simulink model "sim_ES01_03"  (R2021b)
settings: Solver=VariableStepAuto  StartTime=0.0  StopTime=Ts  MaxStep=1e-02  RelTol=1e-3
values from neighbouring files (symbols this model uses):
  c = 2664    [DatiSospensione.m]    (also in Dati_Necessari.m; ES01_Comfort_4dof_stud.m = 0.00047; ES2_2DOF.m = C_values(count2); ES_2DOF_ANIM_TF.m = c_opt)
  k = 35495    [DatiSospensione.m]    (also in Dati_Necessari.m = 99000; ES2_2DOF.m = 99000)
  m = ms+mu    (= 395)    [DatiSospensione.m]    (also in ES01_Comfort_4dof_stud.m = 1790)
  T_sampling = 1/f_sampling    (= 0.001)    [Dati_Necessari.m]    (also in ES_2DOF_ANIM_TF.m)
  Ts = 4    [DatiSospensione.m]    (also in ES_2DOF_ANIM_TF.m = 100)
  z0 = 0    [Dati_Necessari.m]    (also in ES_2DOF_ANIM_TF.m)
  zd0 = 0    [Dati_Necessari.m]    (also in ES_2DOF_ANIM_TF.m)
libraries: simulink x1
settings Model: Creator=Utente  LastModifiedBy=Utente
settings DataIOCC: ReturnWorkspaceOutputs=off

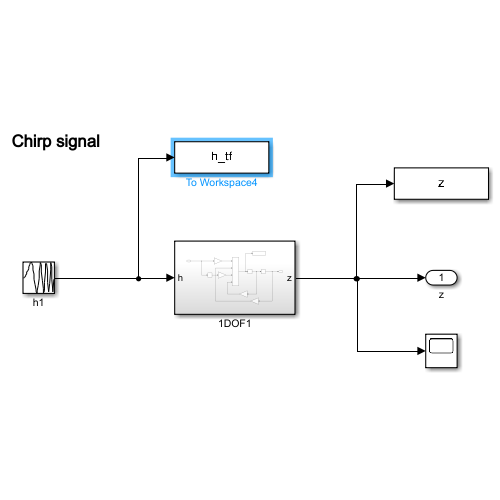
[thumbnail: Simulink's stored preview of the top-level diagram]
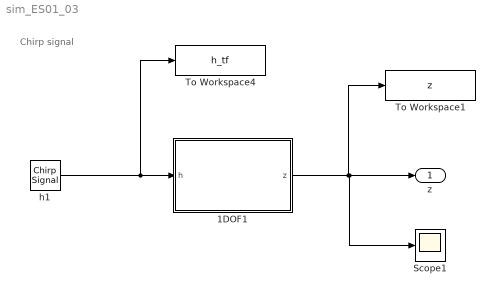
== system sim_ES01_03 ==
  note: Chirp signal
  1DOF1 : Subsystem
  Scope1 : Scope
  To Workspace1 : ToWorkspace  VariableName=z  SaveFormat=Timeseries  SampleTime=1/T_sampling
  To Workspace4 : ToWorkspace  VariableName=h_tf  SaveFormat=Timeseries  SampleTime=1/T_sampling
      settings: Decimation=decimation
  h1 : simulink/Sources/Chirp Signal  f1=w_in  T=Ts  f2=w_end
  z : Outport
  wires:
  h1/1 -> To Workspace4/1, 1DOF1/1(h)
  1DOF1/1(z) -> To Workspace1/1, Scope1/1, z/1

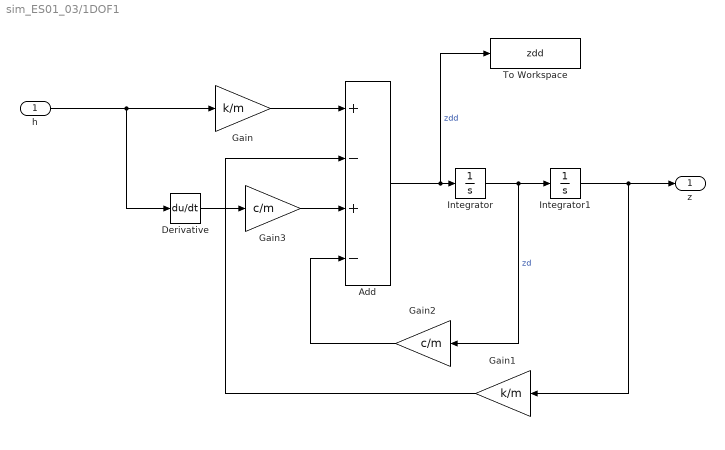
== system sim_ES01_03/1DOF1 ==
  h : Inport
  Add : Sum  Inputs=+-+-
  Derivative : Derivative
  Gain : Gain  Gain=k/m
  Gain1 : Gain  Gain=k/m
  Gain2 : Gain  Gain=c/m
  Gain3 : Gain  Gain=c/m
  Integrator : Integrator  InitialCondition=zd0
  Integrator1 : Integrator  InitialCondition=z0
  To Workspace : ToWorkspace  VariableName=zdd  SaveFormat=Timeseries  SampleTime=1/T_sampling
      settings: Decimation=decimation
  z : Outport
  wires:
  Derivative/1 -> Gain3/1
  Add/1 -> To Workspace/1, Integrator/1  "zdd"
  h/1 -> Derivative/1, Gain/1
  Gain1/1 -> Add/2
  Integrator1/1 -> z/1, Gain1/1
  Gain/1 -> Add/1
  Gain3/1 -> Add/3
  Integrator/1 -> Gain2/1, Integrator1/1  "zd"
  Gain2/1 -> Add/4
